simulink model "provaBderivatieAttitude"  (R2023b)
settings: Solver=VariableStepAuto  StartTime=0.0  StopTime=10.0  RelTol=1e-3
values from neighbouring files (symbols this model uses):
  I = [Ix 0 0; 0 Iy 0; 0 0 Iz]    [gyroscope.m]
  I_inv = inv(I)    [gyroscope.m]
undefined symbols (not defined in the file or in its folder): A, A1, alpha, BODY, c, DCM_eci_per, e, epsilon, Fe, FS, H0, i, inc_tot, j_b, MJD2000_initial, mu_E, n_e, p, pd, ps, q0, r1, r2, r3, R_E, th0, ts_sensor, w0, w_E, w_r
libraries: matrix_library x12, dspindex x3, simulink x1, aerolibutil x1
(part 2 of 2)

== system provaBderivatieAttitude/Dynamics e Kinematics/DCM composition from quaternions 1/Cross product matrix composition ==
  q_vect : Inport
  Demux : Demux  Outputs=3
  Gain : Gain  Gain=[0 0 0; 0 0 -1; 0 1 0]
  Gain1 : Gain  Gain=[0 0 1; 0 0 0; -1 0 0]
  Gain2 : Gain  Gain=[0 -1 0; 1 0 0; 0 0 0]
  Sum : Sum  Inputs=+++
  q_vect cross : Outport
  wires:
  Gain1/1 -> Sum/2
  Demux/3 -> Gain2/1
  Demux/1 -> Gain/1
  q_vect/1 -> Demux/1
  Gain2/1 -> Sum/3
  Demux/2 -> Gain1/1
  Gain/1 -> Sum/1
  Sum/1 -> q_vect cross/1

== system provaBderivatieAttitude/Dynamics e Kinematics/Kinematics quaternion2/Matrix OMEGA ==
  omega : Inport
  Constant4 : Constant  Value=0
  Demux : Demux  Outputs=3
  Gain : Gain  Gain=-1
  Gain1 : Gain  Gain=-1
  Gain2 : Gain  Gain=-1
  Matrix Concatenate : Concatenate  NumInputs=4  Mode=Multidimensional array  ConcatenateDimension=2
  Vector Concatenate{,2..4} (4 alike) : Concatenate  NumInputs=4
  Matrix Omega : Outport
  wires:
  Demux/2 -> Vector Concatenate4/2, Vector Concatenate/3, Gain1/1  "W_v"
  Gain1/1 -> Vector Concatenate2/4, Vector Concatenate3/1
  Matrix Concatenate/1 -> Matrix Omega/1
  Gain2/1 -> Vector Concatenate3/4, Vector Concatenate/2  "-W_w"
  Vector Concatenate3/1 -> Matrix Concatenate/3
  Demux/3 -> Vector Concatenate2/1, Vector Concatenate4/3, Gain2/1  "W_w"
  Gain/1 -> Vector Concatenate/4, Vector Concatenate2/3  "-W_u"
  Constant4/1 -> Vector Concatenate/1, Vector Concatenate2/2, Vector Concatenate3/3, Vector Concatenate4/4
  Demux/1 -> Vector Concatenate3/2, Vector Concatenate4/1, Gain/1  "W_u"
  Vector Concatenate4/1 -> Matrix Concatenate/4
  Vector Concatenate2/1 -> Matrix Concatenate/2
  Vector Concatenate/1 -> Matrix Concatenate/1
  omega/1 -> Demux/1

== system provaBderivatieAttitude/Dynamics e Kinematics/Kinematics quaternion2/Normalize Vector2 ==
  Vector : Inport
  Dot Product : DotProduct  OutDataTypeStr=Inherit: Inherit via internal rule
  Sqrt : Sqrt
  Norm : Outport
  wires:
  Sqrt/1 -> Norm/1
  Vector/1 -> Dot Product/1, Dot Product/2
  Dot Product/1 -> Sqrt/1

== system provaBderivatieAttitude/Subsystem/Normalize Vector3/Normalize Vector ==
  Vector : Inport
  Dot Product : DotProduct  OutDataTypeStr=Inherit: Inherit via internal rule
  Sqrt : Sqrt
  Norm : Outport
  wires:
  Sqrt/1 -> Norm/1
  Vector/1 -> Dot Product/1, Dot Product/2
  Dot Product/1 -> Sqrt/1

== system provaBderivatieAttitude/Subsystem/Normalize Vector4/Normalize Vector ==
  Vector : Inport
  Dot Product : DotProduct  OutDataTypeStr=Inherit: Inherit via internal rule
  Sqrt : Sqrt
  Norm : Outport
  wires:
  Sqrt/1 -> Norm/1
  Vector/1 -> Dot Product/1, Dot Product/2
  Dot Product/1 -> Sqrt/1

== system provaBderivatieAttitude/two-body Keplerian dynamics/Integretion of true anomaly/(1-e^2)^(3//2) ==
  Constant1 : Constant
  Constant2 : Constant  Value=e
  Constant3 : Constant  Value=3/2
  Power : Math  Operator=pow
  Product1 : Product
  Subtract : Sum  Inputs=+-
  Out1 : Outport
  wires:
  Constant3/1 -> Power/2
  Constant2/1 -> Product1/2, Product1/1
  Subtract/1 -> Power/1
  Constant1/1 -> Subtract/1
  Product1/1 -> Subtract/2
  Power/1 -> Out1/1

== system provaBderivatieAttitude/two-body Keplerian dynamics/r_perifocal/Calculation of norm r ==
  th : Inport
  Constant : Constant  Value=p
  Constant2 : Constant
  Cos : Trigonometry  Operator=cos
  Divide : Product  Inputs=*/
  Gain1 : Gain  Gain=e
  Sum : Sum  Inputs=|++
  Norm(r) : Outport
  wires:
  Constant/1 -> Divide/1
  Gain1/1 -> Sum/2
  Constant2/1 -> Sum/1
  Cos/1 -> Gain1/1
  Sum/1 -> Divide/2
  th/1 -> Cos/1
  Divide/1 -> Norm(r)/1

== system provaBderivatieAttitude/Attitude determination algebric Method with 2 sensor/Subsystem/Normalize Vector3/Normalize Vector ==
  Vector : Inport
  Dot Product : DotProduct  OutDataTypeStr=Inherit: Inherit via internal rule
  Sqrt : Sqrt
  Norm : Outport
  wires:
  Sqrt/1 -> Norm/1
  Vector/1 -> Dot Product/1, Dot Product/2
  Dot Product/1 -> Sqrt/1

== system provaBderivatieAttitude/Attitude determination algebric Method with 2 sensor/Subsystem1/Normalize Vector3/Normalize Vector ==
  Vector : Inport
  Dot Product : DotProduct  OutDataTypeStr=Inherit: Inherit via internal rule
  Sqrt : Sqrt
  Norm : Outport
  wires:
  Sqrt/1 -> Norm/1
  Vector/1 -> Dot Product/1, Dot Product/2
  Dot Product/1 -> Sqrt/1

== system provaBderivatieAttitude/Calculation of disturbance torque/M of Solar Pressure/Calculation of F_i/(1-ps)*Sb + (2ps*dot(SB,Nb) +2//3pd))*Ni ==
  body : Inport
  dot(Sb,Nb) : Inport  Port=2
  Sb versor : Inport  Port=3
  Constant5 : Constant  Value=pd
  Gain1 : Gain  Gain=2*ps
  Gain2 : Gain  Gain=2/3
  Gain3 : Gain  Gain=[(A1 - ps) (A1 - ps) (A1 - ps)]
  Matrix Concatenate : Concatenate  NumInputs=3  Mode=Multidimensional array  ConcatenateDimension=2
  Matrix Muly2 : Product
  Sum : Sum  Inputs=|++
  Sum1 : Sum  Inputs=|++
  Out1 : Outport
  wires:
  Sum1/1 -> Matrix Concatenate/1, Matrix Concatenate/3, Matrix Concatenate/2  "2ps*dot(SB,Nb) +2/3pd)"
  Gain1/1 -> Sum1/1
  dot(Sb,Nb)/1 -> Gain1/1
  Gain3/1 -> Sum/2  "(1-ps)*Sb"
  Constant5/1 -> Gain2/1
  Sum/1 -> Out1/1
  Matrix Muly2/1 -> Sum/1  "(2ps*dot(SB,Nb) +2/3pd))*Ni"
  Matrix Concatenate/1 -> Matrix Muly2/2  "Sb_vector"
  Gain2/1 -> Sum1/2
  body/1 -> Matrix Muly2/1
  Sb versor/1 -> Gain3/1

== system provaBderivatieAttitude/Calculation of disturbance torque/M of Solar Pressure/Calculation of F_i/Eliminate effect of face in shadow ==
  dot(SB,Nb) : Inport
  Compare To Zero : simulink/Logic and Bit Operations/Compare To Zero  relop=>=  OutDataTypeStr=boolean
  Product : Product
  dot(SB,Nb)-clean : Outport
  wires:
  dot(SB,Nb)/1 -> Product/2, Compare To Zero/1
  Compare To Zero/1 -> Product/1
  Product/1 -> dot(SB,Nb)-clean/1

== system provaBderivatieAttitude/Calculation of disturbance torque/M of Solar Pressure/Calculation of F_i/Subsystem ==
  dot(SB,Nb) : Inport
  A : Inport  Port=2
  Gain : Gain  Gain=-Fe/c
  Product : Product
  -PA*dot(SB,Nb) : Outport
  wires:
  Product/1 -> Gain/1
  A/1 -> Product/2
  Gain/1 -> -PA*dot(SB,Nb)/1  "-PA*dot(SB,Nb)"
  dot(SB,Nb)/1 -> Product/1

== system provaBderivatieAttitude/Calculation of disturbance torque/M of Solar Pressure/Calculation of F_i/dot(Sb,Nb) ==
  body versor matrix : Inport
  Sb_vector1 : Inport  Port=2
  Constant2 : Constant  Value=ones(length(BODY),1)  VectorParams1D=off
  Matrix Multiply : Product  Multiplication=Matrix(*)
  Matrix Muly1 : Product
  Sum of Elements : Sum  Inputs=+  CollapseMode=Specified dimension  CollapseDim=2
  Transpose : Math  Operator=transpose
  dot(SB,Nb) : Outport
  Sb_matrix : Outport  Port=2
  wires:
  Matrix Muly1/1 -> Sum of Elements/1
  Matrix Multiply/1 -> Sb_matrix/1, Matrix Muly1/2  "Sb_vector"
  Constant2/1 -> Matrix Multiply/1
  Sb_vector1/1 -> Transpose/1
  body versor matrix/1 -> Matrix Muly1/1
  Sum of Elements/1 -> dot(SB,Nb)/1  "dot(SB,Nb)"
  Transpose/1 -> Matrix Multiply/2

== system provaBderivatieAttitude/Calculation of disturbance torque/M of Solar Pressure/Normalize Vector/Normalize Vector ==
  Vector : Inport
  Dot Product : DotProduct  OutDataTypeStr=Inherit: Inherit via internal rule
  Sqrt : Sqrt
  Norm : Outport
  wires:
  Sqrt/1 -> Norm/1
  Vector/1 -> Dot Product/1, Dot Product/2
  Dot Product/1 -> Sqrt/1

== system provaBderivatieAttitude/Calculation of disturbance torque/M of Solar Pressure/Torque calculation/Subsystem ==
  a2 : Inport
  a3 : Inport  Port=2
  Gain : Gain  Gain=r3
  Gain1 : Gain  Gain=r2
  Subtract : Sum  Inputs=+-
  M_i : Outport
  wires:
  a2/1 -> Gain/1
  a3/1 -> Gain1/1
  Gain/1 -> Subtract/1
  Gain1/1 -> Subtract/2
  Subtract/1 -> M_i/1

== system provaBderivatieAttitude/Calculation of disturbance torque/M of Solar Pressure/Torque calculation/Subsystem1 ==
  a3 : Inport
  a1 : Inport  Port=2
  Gain : Gain  Gain=r1
  Gain1 : Gain  Gain=r3
  Subtract : Sum  Inputs=+-
  M_j : Outport
  wires:
  a3/1 -> Gain/1
  a1/1 -> Gain1/1
  Gain/1 -> Subtract/1
  Gain1/1 -> Subtract/2
  Subtract/1 -> M_j/1

== system provaBderivatieAttitude/Calculation of disturbance torque/M of Solar Pressure/Torque calculation/Subsystem2 ==
  a1 : Inport
  a2 : Inport  Port=2
  Gain : Gain  Gain=r2
  Gain1 : Gain  Gain=r1
  Subtract : Sum  Inputs=+-
  M_i : Outport
  wires:
  a1/1 -> Gain/1
  a2/1 -> Gain1/1
  Gain/1 -> Subtract/1
  Gain1/1 -> Subtract/2
  Subtract/1 -> M_i/1

== system provaBderivatieAttitude/Dipol Model of Magnetic Field/Calculation of b_n/Normalize Vector/Normalize Vector1 ==
  Vector : Inport
  Dot Product : DotProduct  OutDataTypeStr=Inherit: Inherit via internal rule
  Sqrt : Sqrt
  Norm : Outport
  wires:
  Sqrt/1 -> Norm/1
  Vector/1 -> Dot Product/1, Dot Product/2
  Dot Product/1 -> Sqrt/1

== matlab function provaBderivatieAttitude/Sun Position in Earth Centred Equatorial Inertial RF/MATLAB Function1 ==
  data: MJD2000 input; r output
function r = fcn(MJD2000)
     [kep, mu_S] = uplanet(MJD2000, 3); % important that in uplanet there is an initialisation of kep like kep = zeros(6,1);
     r = kep2carRAD(kep, mu_S);
end

== matlab function provaBderivatieAttitude/Statistical methods attitude determination (quaternion  Wabha’s problem) /Blocco da convertire in formato simulink. Ho trovato 3 soluzioni differenti al proble ==
  data: K input; q output; S input; Sadj input
function q = fcn(K, S, Sadj)
    
    A = eig(K);
    A = real(A);
    lambda = max(A);
    z = K(1:3, 4);

    %{
    FUNZIONAAA
    %proposta wikipedia
    sigma = 1/2*trace(S);
    %Sadj = det(S)*eye(3)*inv(S);
    k = trace(Sadj);
    delta = det(S);
    alpha = lambda^2 - sigma^2 + k;
    beta = lambda - sigma;
    gamma = (lambda + sigma)*alpha - delta;
    
    x = (alpha*eye(3) + beta*S + S^2)*z;
    
    q =[x; gamma]/sqrt(gamma^2 + norm(x)^2);
    %}
   
    %
    %Proposta libro: FUNZIONAAAAAA -> sceglierei questa: è facile da
    %implementare
    
    z = K(1:3, 4);
    sigma = K(4,4);
    
    mat = (lambda + sigma)*eye(3) - S;
    q = zeros(4,1);
    q(1:3) = (det(mat)*eye(3)*inv(mat)) * z;
    q(4) = det(mat);
    q = q/norm(q);
    %}


    %{
    GIUSTA FUNZIONA, ma restituisce gibbs vector
    z = K(1:3, 4);
    sigma = K(4,4);
    %K = K - eye(4)*lambda;
    
    % linear system
    %Z = zeros(4,1);
    %q = K\Z;
    %q = q/norm(q);
    
    g = (S-(sigma+lambda)*eye(3)) \ (-z);
    
    DCM = [1+g(1)^2-g(2)^2-g(3)^2, 2*(g(1)*g(2)+g(3))    ,  2*(g(1)*g(3)-g(2));
         2*(g(1)*g(2)-g(3))    , 1-g(1)^2+g(2)^2-g(3)^2,  2*(g(2)*g(3)+g(1));
         2*(g(1)*g(3)+g(2))    , 2*(g(2)*g(3)-g(1))    ,  1-g(1)^2-g(2)^2+g(3)^2];
    DCM = DCM./(1+g(1)^2+g(2)^2+g(3)^2);
    %}

    %{
    % soluzione nelle slide, ma la matrice è singolare
    q = (K - lambda*eye(4)) \ zeros(4,1);
    q = q/norm(q);
    %}

end

== matlab function provaBderivatieAttitude/Ouput DCM with gibbs vector (ver slide) ==
  data: alpha input; DCM output; s input; v input
function DCM = fcn(alpha, s, v)

B = zeros(3,3);
K = zeros(4,4);
%
for i = 1:size(s,2)
    B = B + alpha(i)*s(:,i)*v(:,i)';
end

S = B' + B;

z = [B(2,3) - B(3,2), B(3,1) - B(1,3), B(1,2) - B(2,1)]';
sigma = trace(B);
K(1:3, 1:3) = S-eye(3,3)*sigma;
K(1:3,4) = z;
K(4, 1:3) = z';
K(4,4) = sigma;

A = eig(K);
A = real(A);
lambda = max(A);
%K = K - eye(4)*lambda;

% linear system
%Z = zeros(4,1);
%q = K\Z;
%q = q/norm(q);

g = (S-(sigma+lambda)*eye(3)) \ (-z);

DCM = [1+g(1)^2-g(2)^2-g(3)^2, 2*(g(1)*g(2)+g(3))    ,  2*(g(1)*g(3)-g(2));
     2*(g(1)*g(2)-g(3))    , 1-g(1)^2+g(2)^2-g(3)^2,  2*(g(2)*g(3)+g(1));
     2*(g(1)*g(3)+g(2))    , 2*(g(2)*g(3)-g(1))    ,  1-g(1)^2-g(2)^2+g(3)^2];
DCM = DCM./(1+g(1)^2+g(2)^2+g(3)^2);

end
